simulink model "Simple_Subsys_MR"  (R2018b)
settings: Solver=VariableStepAuto  StartTime=0.0  StopTime=10.0  RelTol=1e-3
settings Model: Creator=Rose  LastModifiedBy=Rose
settings OptimizationCC: DefaultParameterBehavior=Inlined
settings DebuggingCC: LibraryContextMissingDiagnostic=none
settings SFSimCC: SimUseLocalCustomCode=off
settings RTWCC: RTWUseLocalCustomCode=off

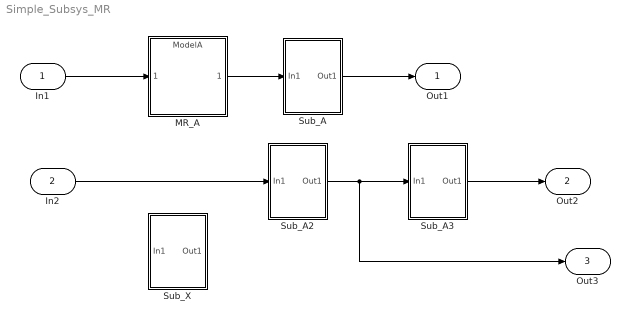
== system Simple_Subsys_MR ==
  In1 : Inport  OutDataTypeStr=double
  In2 : Inport  Port=2  OutDataTypeStr=double
  MR_A : ModelReference  ModelNameDialog=ModelA  SimulationMode=Normal  ModelReferenceVersion=1.4
  Sub_A : Subsystem
  Sub_A2 : Subsystem
  Sub_A3 : Subsystem
  Sub_X : Subsystem
  Out1 : Outport  OutDataTypeStr=double
  Out2 : Outport  Port=2  OutDataTypeStr=double
  Out3 : Outport  Port=3  OutDataTypeStr=double
  wires:
  In1/1 -> MR_A/1
  MR_A/1 -> Sub_A/1(In1)
  Sub_A/1(Out1) -> Out1/1
  In2/1 -> Sub_A2/1(In1)
  Sub_A2/1(Out1) -> Out3/1, Sub_A3/1(In1)
  Sub_A3/1(Out1) -> Out2/1

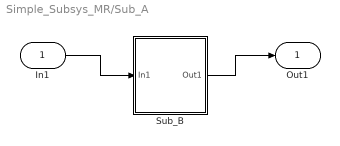
== system Simple_Subsys_MR/Sub_A ==
  In1 : Inport  OutDataTypeStr=double
  Sub_B : Subsystem
  Out1 : Outport  OutDataTypeStr=double
  wires:
  Sub_B/1(Out1) -> Out1/1
  In1/1 -> Sub_B/1(In1)

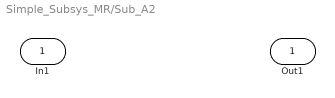
== system Simple_Subsys_MR/Sub_A2 ==
  In1 : Inport  OutDataTypeStr=double
  Out1 : Outport  OutDataTypeStr=double

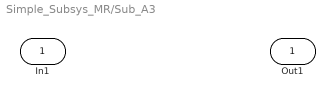
== system Simple_Subsys_MR/Sub_A3 ==
  In1 : Inport  OutDataTypeStr=double
  Out1 : Outport  OutDataTypeStr=double

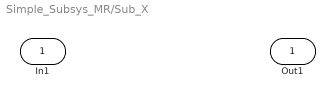
== system Simple_Subsys_MR/Sub_X ==
  In1 : Inport  OutDataTypeStr=double
  Out1 : Outport  OutDataTypeStr=double

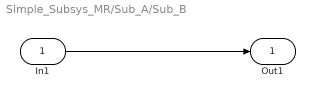
== system Simple_Subsys_MR/Sub_A/Sub_B ==
  In1 : Inport  OutDataTypeStr=double
  Out1 : Outport  OutDataTypeStr=double
  wires:
  In1/1 -> Out1/1
